simulink model "Ciclo_Aperto"  (R2019b)
settings: Solver=VariableStepAuto  StartTime=0.0  StopTime=tf  RelTol=1e-3
values from neighbouring files (symbols this model uses):
  A = [ ... (first row only)    [main.m]
  B = [ ... (first row only)    [main.m]
  C = [0 0 1]    [main.m]
  D = 0    [main.m]
  x0 = [0 0 deg*pi/180]'    [main.m]
settings Model: Creator=giuliorusso  LastModifiedBy=giuliorusso

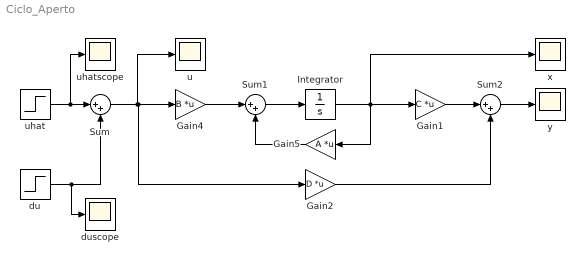
== system Ciclo_Aperto ==
  Gain1 : Gain  Gain=C  Multiplication=Matrix(K*u)
  Gain2 : Gain  Gain=D  Multiplication=Matrix(K*u)
  Gain4 : Gain  Gain=B  Multiplication=Matrix(K*u)
  Gain5 : Gain  Gain=A  Multiplication=Matrix(K*u)
  Integrator : Integrator  InitialCondition=x0
  Sum : Sum  Inputs=|++
  Sum1 : Sum  Inputs=|++
  Sum2 : Sum  Inputs=|++
  du : Step  Time=3  Before=1.5  After=0  SampleTime=0
  duscope : Scope
  u : Scope
  uhat : Step  Time=0  After=0  SampleTime=0
  uhatscope : Scope
  x : Scope
  y : Scope
  wires:
  Integrator/1 -> x/1, Gain5/1, Gain1/1
  Sum1/1 -> Integrator/1
  Gain5/1 -> Sum1/2
  Gain4/1 -> Sum1/1
  Gain2/1 -> Sum2/2
  Gain1/1 -> Sum2/1
  Sum2/1 -> y/1
  du/1 -> duscope/1, Sum/2
  Sum/1 -> u/1, Gain2/1, Gain4/1
  uhat/1 -> uhatscope/1, Sum/1
